simulink model "AYBfinal"  (R2023a)
settings: Solver=VariableStepAuto  StartTime=0.0  StopTime=5  RelTol=1e-3
libraries: spsFourierLib x7, spsMultimeterLib x6, spsParallelRLCBranchLib x4, spsPowerLib x4, spsSeriesRLCBranchLib x4, spsACVoltageSourceLib x3, spsCurrentMeasurementLib x3, spsLinearTransformerLib x3, spsVoltageMeasurementLib x1, sps_lib x1
settings Model: Creator=Pablo Gutierrez  LastModifiedBy=USUARIO
settings OptimizationCC: ReuseModelBlockBuffer=off

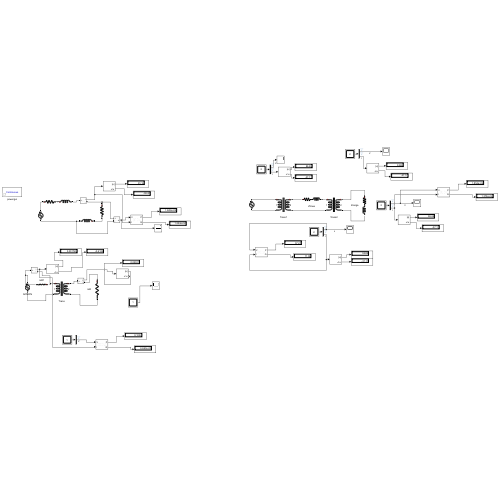
[thumbnail: Simulink's stored preview of the top-level diagram]
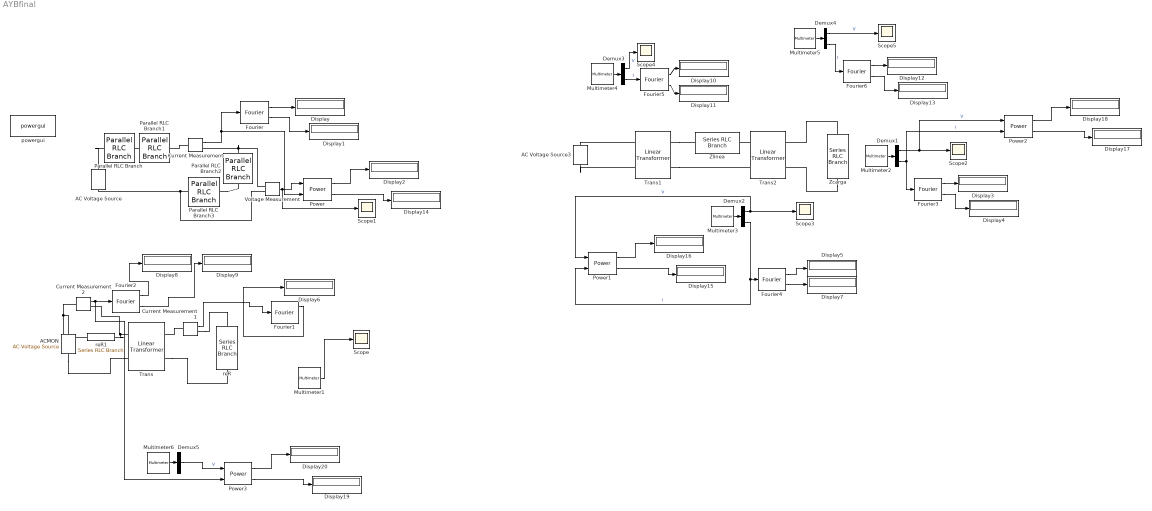
== system AYBfinal ==
  AC Voltage Source : spsACVoltageSourceLib/AC Voltage Source  Amplitude=480  Phase=0  Frequency=60  SampleTime=0  Measurements=None  BusType=swing  Pref=10e3  Qref=0  Qmin=-inf  Qmax=+inf
  AC Voltage Source3 : spsACVoltageSourceLib/AC Voltage Source  Amplitude=480  Phase=0  Frequency=60  SampleTime=0  Measurements=None  BusType=swing  Pref=10e3  Qref=0  Qmin=-inf  Qmax=+inf
  ACMON : spsACVoltageSourceLib/AC Voltage Source  Amplitude=120  Phase=0  Frequency=60  SampleTime=0  Measurements=Voltage  BusType=swing  Pref=10e3  Qref=0  Qmin=-inf  Qmax=+inf
  Current Measurement : spsCurrentMeasurementLib/Current Measurement  PhasorSimulation=off  OutputType=Complex  PSBequivalent=0
  Current Measurement1 : spsCurrentMeasurementLib/Current Measurement  PhasorSimulation=off  OutputType=Complex  PSBequivalent=0
  Current Measurement2 : spsCurrentMeasurementLib/Current Measurement  PhasorSimulation=off  OutputType=Complex  PSBequivalent=0
  Demux{1..4} (4 alike) : Demux  Outputs=2
  Demux5 : Demux  Outputs=1
  Display{,1..20} (21 alike) : Display
  Fourier{,1..6} (7 alike) : spsFourierLib/Fourier  Freq=60  n=1  InInit=[0, 0]  Ts=0
  Multimeter1 : spsMultimeterLib/Multimeter  L=29  sel=3  yselected={}  Gain=1  OutputType=Complex  PlotAtSimulationStop=off  PhasorSimulation=off
  Multimeter2 : spsMultimeterLib/Multimeter  L=29  sel=[1 13]  yselected={}  Gain=[1 1]  OutputType=Complex  PlotAtSimulationStop=off  PhasorSimulation=off
  Multimeter3 : spsMultimeterLib/Multimeter  L=29  sel=[2 14]  yselected={}  Gain=[1 1]  OutputType=Complex  PlotAtSimulationStop=off  PhasorSimulation=off
  Multimeter4 : spsMultimeterLib/Multimeter  L=29  sel=[8 20]  yselected={}  Gain=[1 1]  OutputType=Complex  PlotAtSimulationStop=off  PhasorSimulation=off
  Multimeter5 : spsMultimeterLib/Multimeter  L=29  sel=[10 22]  yselected={}  Gain=[1 1]  OutputType=Complex  PlotAtSimulationStop=off  PhasorSimulation=off
  Multimeter6 : spsMultimeterLib/Multimeter  L=29  sel=12  yselected={}  Gain=1  OutputType=Complex  PlotAtSimulationStop=off  PhasorSimulation=off
  Parallel RLC Branch : spsParallelRLCBranchLib/Parallel RLC Branch  LConnTagsString=a  RConnTagsString=__new0  BranchType=R  Resistance=0.18  Inductance=1e-3  SetiL0=off  InitialCurrent=0  Capacitance=1e-6  Setx0=off  InitialVoltage=0  Measurements=Branch voltage and current
  Parallel RLC Branch1 : spsParallelRLCBranchLib/Parallel RLC Branch  LConnTagsString=a  RConnTagsString=__new0  BranchType=L  Resistance=1  Inductance=0.28/(2*pi*60)  SetiL0=off  InitialCurrent=0  Capacitance=1e-6  Setx0=off  InitialVoltage=0  Measurements=Branch voltage and current
  Parallel RLC Branch2 : spsParallelRLCBranchLib/Parallel RLC Branch  LConnTagsString=a  RConnTagsString=__new0  BranchType=R  Resistance=4  Inductance=1e-3  SetiL0=off  InitialCurrent=0  Capacitance=1e-6  Setx0=off  InitialVoltage=0  Measurements=Branch voltage and current
  Parallel RLC Branch3 : spsParallelRLCBranchLib/Parallel RLC Branch  LConnTagsString=a  RConnTagsString=__new0  BranchType=L  Resistance=1  Inductance=3/(2*pi*60)  SetiL0=off  InitialCurrent=0  Capacitance=1e-6  Setx0=off  InitialVoltage=0  Measurements=Branch current
  Power{,1..3} (4 alike) : spsPowerLib/Power  Freq=60  Vinit=[1, 0]  Iinit=[1, 0]  Ts=0
  Scope{,1..5} (6 alike) : Scope
  Trans : spsLinearTransformerLib/Linear Transformer  UNITS=SI  NominalPower=[ 250e6 60 ]  winding1=[120 0 0]  winding2=[9 0 0]  ThreeWindings=off  winding3=[3.15e+05 0.7938 0.084225]  RmLm=[1.0804e+10 286600]  Measurements=None  DataType=on
  Trans1 : spsLinearTransformerLib/Linear Transformer  UNITS=SI  NominalPower=[ 250e6 60 ]  winding1=[480 0 0]  winding2=[480*10 0 0]  ThreeWindings=off  winding3=[3.15e+05 0.7938 0.084225]  RmLm=[1.0804e+10 286600]  Measurements=All voltages and currents  DataType=on
  Trans2 : spsLinearTransformerLib/Linear Transformer  UNITS=SI  NominalPower=[ 250e6 60 ]  winding1=[480*10 0 0]  winding2=[480 0 0]  ThreeWindings=off  winding3=[3.15e+05 0.7938 0.084225]  RmLm=[1.0804e+10 286600]  Measurements=All voltages and currents  DataType=on
  Voltage Measurement : spsVoltageMeasurementLib/Voltage Measurement  PhasorSimulation=off  OutputType=Complex  PSBequivalent=0
  Zcarga : spsSeriesRLCBranchLib/Series RLC Branch  LConnTagsString=__new0  RConnTagsString=__new0  BranchType=RL  Resistance=4  Inductance=0.00796  SetiL0=off  InitialCurrent=0  Capacitance=0  Setx0=off  InitialVoltage=0  Measurements=Branch voltage and current
  Zlinea : spsSeriesRLCBranchLib/Series RLC Branch  LConnTagsString=__new0  RConnTagsString=__new0  BranchType=RL  Resistance=0.8  Inductance=0.00064  SetiL0=off  InitialCurrent=0  Capacitance=0  Setx0=off  InitialVoltage=0  Measurements=Branch voltage and current
  powergui : sps_lib/powergui  Priority=1  SimulationMode=Continuous  SampleTime=50e-6  frequency=60  Iterations=50  frequencyindice=60  Pbase=100e6  ErrMax=1e-4  UnitsV=kV  UnitsW=MW  buscounter=0  FunctionMessages=off  echomessages=off  EnableUseOfTLC=off  CurrentSourceSwitches=off  DisableSnubberDevices=off  DisableRonSwitches=off  DisableVfSwitches=off  DisplayEquations=off  AutomaticDiscreteSolvers=off  SolverType=Tustin/Backward Euler (TBE)  Interpol=off  ExternalGateDelay=off  methode=off  Ts=100  x0status=blocks  SPID=on  SwTol=0  HookPort=off  NonlinearTolerance=1e-4  nMaxIteration=100  ContinueOnMaxIteration=off  RestoreLinks=warning  ResistiveCurrentMeasurement=off  Frange=[0:2:500]  Ylog=off  Xlog=on  ShowGrid=off  save=off  variable=ZData  structure=0  ZoomFFT=off  StartTime=0.0  cycles=1  DisplayStyle=1  fundamental=60  FreqAxis=off  MaxFrequency=1000  frequencyindicesteady=1  RmsSteady=1  display=off
  reR : spsSeriesRLCBranchLib/Series RLC Branch  LConnTagsString=__new0  RConnTagsString=__new0  BranchType=R  Resistance=390  Inductance=1e-3  SetiL0=off  InitialCurrent=0  Capacitance=0  Setx0=off  InitialVoltage=0  Measurements=Branch voltage
  reR1 : spsSeriesRLCBranchLib/Series RLC Branch  LConnTagsString=__new0  RConnTagsString=__new0  BranchType=R  Resistance=1.8  Inductance=1e-3  SetiL0=off  InitialCurrent=0  Capacitance=0  Setx0=off  InitialVoltage=0  Measurements=Branch voltage and current
  wires:
  Current Measurement/1 -> Power/2, Fourier/1
  Fourier/1 -> Display/1
  Fourier/2 -> Display1/1
  Voltage Measurement/1 -> Scope1/1, Power/1
  Power/1 -> Display2/1
  Current Measurement1/1 -> Fourier1/1
  Fourier1/1 -> Display6/1
  Fourier2/2 -> Display9/1
  Fourier2/1 -> Display8/1
  Current Measurement2/1 -> Power3/2, Fourier2/1
  Multimeter1/1 -> Scope/1
  Demux1/2 -> Fourier3/1, Power2/2  "I"
  Demux1/1 -> Power2/1, Scope2/1  "V"
  Multimeter2/1 -> Demux1/1
  Fourier3/1 -> Display3/1
  Fourier3/2 -> Display4/1
  Fourier4/1 -> Display5/1
  Fourier4/2 -> Display7/1
  Demux2/1 -> Power1/1, Scope3/1  "V"
  Multimeter3/1 -> Demux2/1
  Demux2/2 -> Power1/2, Fourier4/1  "I"
  Demux3/1 -> Scope4/1  "V"
  Demux3/2 -> Fourier5/1  "I"
  Fourier5/1 -> Display10/1
  Multimeter4/1 -> Demux3/1
  Fourier5/2 -> Display11/1
  Demux4/1 -> Scope5/1  "V"
  Demux4/2 -> Fourier6/1  "I"
  Fourier6/1 -> Display12/1
  Multimeter5/1 -> Demux4/1
  Fourier6/2 -> Display13/1
  Power/2 -> Display14/1
  Power1/2 -> Display15/1
  Power1/1 -> Display16/1
  Power2/2 -> Display17/1
  Power2/1 -> Display18/1
  Power3/2 -> Display19/1
  Power3/1 -> Display20/1
  Multimeter6/1 -> Demux5/1
  Demux5/1 -> Power3/1  "V"
  connections:
  Parallel RLC Branch/RConn1 -- Parallel RLC Branch1/LConn1
  Parallel RLC Branch/LConn1 -- AC Voltage Source/RConn1
  Parallel RLC Branch3/RConn1 -- Voltage Measurement/LConn2 -- AC Voltage Source/LConn1
  Parallel RLC Branch3/LConn1 -- Parallel RLC Branch2/RConn1
  Parallel RLC Branch2/LConn1 -- Current Measurement/RConn1 -- Voltage Measurement/LConn1
  Current Measurement/LConn1 -- Parallel RLC Branch1/RConn1
  ACMON/LConn1 -- Trans/LConn2
  Trans/RConn2 -- reR/RConn1
  Current Measurement1/RConn1 -- reR/LConn1
  Current Measurement1/LConn1 -- Trans/RConn1
  Trans1/RConn1 -- Zlinea/LConn1
  Trans1/LConn1 -- AC Voltage Source3/RConn1
  AC Voltage Source3/LConn1 -- Trans1/LConn2
  Trans2/LConn1 -- Zlinea/RConn1
  Trans1/RConn2 -- Trans2/LConn2
  Zcarga/LConn1 -- Trans2/RConn1
  Zcarga/RConn1 -- Trans2/RConn2
  ACMON/RConn1 -- reR1/RConn1 -- Current Measurement2/LConn1
  Trans/LConn1 -- reR1/LConn1 -- Current Measurement2/RConn1
